simulink model "RobotX_ss_acousticsSingle_Dock_LB_ODOA_T_1024_NewLidarMode"  (R2014a)
settings: Solver=FixedStepDiscrete  StartTime=0.0  StopTime=inf  FixedStep=.25  RelTol=1e-3
undefined symbols (not defined in the file): Com1, Com2, Com3, Com4, DiscIntNeverNeededParam, standard
libraries: xpcseriallib x42, simulink x19, slrtlib x7, dspmtrx3 x2, speedgoatlib x2, speedgoatlib_IO102 x1
(part 4 of 7)

== matlab function RobotX_ss_acousticsSingle_Dock_LB_ODOA_T_1024_NewLidarMode/Main FSM/Start//Speedgate/Aim/LLA to NED ==
  data: LLA input; GoalNED output; NED_origin input
function GoalNED = LLA2NEDfun(LLA,NED_origin)
%Written by Anderson Lebbad on September 20, 2014
%Last edited by:
%
%This function converts a target Latitude, Longitude, Altitude (LLA) point
%into North, East, Down (NED) coordinates

%First convert to earth centered, earth fixed frame
GoalECEF = lla2ecef([LLA*(pi/180), 0]');
%Then convert from ECEF to North East Down
GoalNEDvect = ecef2ned(NED_origin'*(pi/180),GoalECEF);
GoalNED = GoalNEDvect(1:2)';


end

function x_ecef = lla2ecef(x_lla)
% LLE2ECEF: Converts from geodetic latitude, longitude, and altitude to earth-centered earth-fixed Cartesian coordinates
% INPUT: latitude phi (rad), longitude lambda (rad), altitude h (m)
% OUTPUT: [x, y, z]' (m) earth-centered earth-fixed Cartesian coordinates
    a = 6378137; % equatorial radius of ellipsoid (semi-major axis) (m)
    b = 6356752; % polar axis radius of ellipsoid (semi-minor axis) (m)

    phi = x_lla(1);
    lambda = x_lla(2);
    h = x_lla(3);
    
    % auxiliar quantities f, e, and N
    f = (a-b)/a;
    e = f*(2-f);
    N = a/sqrt(1-(e*sin(phi))^2);
    x_ecef = [(N+h)*cos(phi)*cos(lambda); (N+h)*cos(phi)*sin(lambda); (N*(1-e^2)+h)*sin(phi)];
end

function [x_ned] = ecef2ned(ned_lla, x_ecef)
% ECEF2NED Converts from earth-centered, earth-fixed Cartesian coordinates to tangent plane
% INPUT:
% 1) x_ecef=[x,y,z]' (m) earth-centered, earth-fixed Cartesian coordinates
% 2) ned_lla=[phi,lambda]' consiting of latitude phi (rad), longitude lambda (rad) of NED origin
% OUTPUT:
% 1) x_ned=[x,y,z]' (m) in NED coordinate system with the origin [phi,lambda]'

    phi = ned_lla(1);
    lambda = ned_lla(2);

    % transformation  matrix
    T = [-sin(phi)*cos(lambda) -sin(phi)*sin(lambda)  cos(phi)
         -sin(lambda)           cos(lambda)           0
          cos(phi)*cos(lambda)   cos(phi)*sin(lambda)  sin(phi)];

     x_ned = T*(x_ecef-lla2ecef([phi, lambda, 0]')); % convert to NED
     x_ned(3) = -x_ned(3);
end

== matlab function RobotX_ss_acousticsSingle_Dock_LB_ODOA_T_1024_NewLidarMode/Main FSM/Termination/CalcTimes ==
  data: pts input; u input; Data output
function Data = calcTimes(pts, u)
%Written by Anderson Lebbad on August 9, 2014
%Last Edited: Dylan DeGaetano September 1, 2014

%Calculates times for the boat to get to points for a trajectory, and
%formats Data for communication

%Initialize
Data = zeros(24,1);
traj = zeros(8,3);
traj(:,1:2) = pts;



for k = 2:8
    %Calculate distance to travel from last point
    distTravel = sqrt(sum((pts(k-1,:)-pts(k,:)).^2));
    %Assume 1m per second speed
    traj(k,3) = traj(k-1,3) + distTravel;
    %Add time based off initial velocity to get to first point past initial
    if k == 2
        traj(k,3) = traj(k,3) + 2.5*abs(2-u);
    end
end


%Output Data
for i=1:8
    for j = 1:3
        Data(3*(i-1)+j) = traj(i,j);
    end
end

== matlab function RobotX_ss_acousticsSingle_Dock_LB_ODOA_T_1024_NewLidarMode/Main FSM/Termination/LLA to NED ==
  data: Course input; GoalLLA input; GoalNED output; NED_origin input
function GoalNED = LLA2NEDfun(Course,GoalLLA,NED_origin)
%Written by Anderson Lebbad on September 20, 2014
%Last edited by:
%
%This function converts a target Latitude, Longitude, Altitude (LLA) point
%into North, East, Down (NED) coordinates

%First convert to earth centered, earth fixed frame
GoalECEF1 = lla2ecef([GoalLLA(1,:)*(pi/180), 0]');
%Then convert from ECEF to North East Down
GoalNEDvect1 = ecef2ned(NED_origin'*(pi/180),GoalECEF1);
GoalNED1 = GoalNEDvect1(1:2)';

%First convert to earth centered, earth fixed frame
GoalECEF2 = lla2ecef([GoalLLA(2,:)*(pi/180), 0]');
%Then convert from ECEF to North East Down
GoalNEDvect2 = ecef2ned(NED_origin'*(pi/180),GoalECEF2);
GoalNED2 = GoalNEDvect2(1:2)';

GoalNED = (GoalNED1 + GoalNED2) / 2;

if Course == uint8('T')
    GoalNED = GoalLLA(1,:);
end

end

function x_ecef = lla2ecef(x_lla)
% LLE2ECEF: Converts from geodetic latitude, longitude, and altitude to earth-centered earth-fixed Cartesian coordinates
% INPUT: latitude phi (rad), longitude lambda (rad), altitude h (m)
% OUTPUT: [x, y, z]' (m) earth-centered earth-fixed Cartesian coordinates
    a = 6378137; % equatorial radius of ellipsoid (semi-major axis) (m)
    b = 6356752; % polar axis radius of ellipsoid (semi-minor axis) (m)

    phi = x_lla(1);
    lambda = x_lla(2);
    h = x_lla(3);
    
    % auxiliar quantities f, e, and N
    f = (a-b)/a;
    e = f*(2-f);
    N = a/sqrt(1-(e*sin(phi))^2);
    x_ecef = [(N+h)*cos(phi)*cos(lambda); (N+h)*cos(phi)*sin(lambda); (N*(1-e^2)+h)*sin(phi)];
end

function [x_ned] = ecef2ned(ned_lla, x_ecef)
% ECEF2NED Converts from earth-centered, earth-fixed Cartesian coordinates to tangent plane
% INPUT:
% 1) x_ecef=[x,y,z]' (m) earth-centered, earth-fixed Cartesian coordinates
% 2) ned_lla=[phi,lambda]' consiting of latitude phi (rad), longitude lambda (rad) of NED origin
% OUTPUT:
% 1) x_ned=[x,y,z]' (m) in NED coordinate system with the origin [phi,lambda]'

    phi = ned_lla(1);
    lambda = ned_lla(2);

    % transformation  matrix
    T = [-sin(phi)*cos(lambda) -sin(phi)*sin(lambda)  cos(phi)
         -sin(lambda)           cos(lambda)           0
          cos(phi)*cos(lambda)   cos(phi)*sin(lambda)  sin(phi)];

     x_ned = T*(x_ecef-lla2ecef([phi, lambda, 0]')); % convert to NED
     x_ned(3) = -x_ned(3);
end

== system RobotX_ss_acousticsSingle_Dock_LB_ODOA_T_1024_NewLidarMode/Sensors/1020 Comms/ Raspberry Pi LCM (Navigation) ==
  LCM Input : Inport
  ASCII Decode 6 : xpcseriallib/ASCII Decode   format=P1:%f P2:%f P3:%f V1:%f V2:%f V3:%f E1:%f E2:%f E3:%f Lat:%f Long:%f Pt1:%f Pt2:%f St1:%f St2:%f Start:%f Elapsed:%f RC:%d Deploy:%u Elapsed:%f Bearing1:%f Bearing2:%f Range:%f X_Pos:%f Y_Pos:%f \r\n  nvars=25  vartypes={}
  Bus Creator1 : BusCreator  Inputs=3
  Bus Creator2 : BusCreator  Inputs=3
  Bus Creator3 : BusCreator  Inputs=3
  Bus Creator4 : BusCreator  Inputs=9
  Bus Creator5 : BusCreator  Inputs=2
  Bus Creator6 : BusCreator  Inputs=2
  Bus Creator7 : BusCreator  Inputs=2
  Bus Creator8 : BusCreator  Inputs=7
  Data Type Conversion : DataTypeConversion  OutDataTypeStr=double
  FIFO ASCII read 1 : xpcseriallib/FIFO ASCII read   header={'P1:'}  term=[13 10]  hold=Zero output if no new data  enable=off  maxsize=2000  outputtype=8 bit uint null terminated  sampletime=-1
  LCM Output : Outport
  Acou LCM : Outport  Port=2
  wires:
  LCM Input/1 -> FIFO ASCII read 1/1
  FIFO ASCII read 1/1 -> ASCII Decode 6/1
  Bus Creator4/1 -> LCM Output/1  "Navigation Message"
  ASCII Decode 6/1 -> Bus Creator1/1  "X"
  ASCII Decode 6/2 -> Bus Creator1/2  "Y"
  ASCII Decode 6/3 -> Bus Creator1/3  "Psi"
  Bus Creator1/1 -> Bus Creator4/1  "Pose"
  ASCII Decode 6/4 -> Bus Creator2/1  "u"
  ASCII Decode 6/5 -> Bus Creator2/2  "v"
  Bus Creator2/1 -> Bus Creator4/2  "Velocity"
  ASCII Decode 6/7 -> Bus Creator3/1  "Roll"
  ASCII Decode 6/8 -> Bus Creator3/2  "Pitch"
  ASCII Decode 6/9 -> Bus Creator3/3  "Yaw"
  Bus Creator3/1 -> Bus Creator4/3  "Euler"
  Bus Creator5/1 -> Bus Creator4/5  "Port"
  Bus Creator6/1 -> Bus Creator4/6  "Stbd"
  ASCII Decode 6/14 -> Bus Creator6/1  "StThrust"
  ASCII Decode 6/15 -> Bus Creator6/2  "StAzimuth"
  ASCII Decode 6/12 -> Bus Creator5/1  "PtThrust"
  ASCII Decode 6/13 -> Bus Creator5/2  "PtAzimuth"
  ASCII Decode 6/16 -> Bus Creator4/7  "Start"
  ASCII Decode 6/17 -> Bus Creator4/8  "Elapsed"
  ASCII Decode 6/18 -> Data Type Conversion/1  "On/Off/RC/Auto"
  Data Type Conversion/1 -> Bus Creator4/9  "On/Off/RC/Auto"
  ASCII Decode 6/6 -> Bus Creator2/3  "r"
  ASCII Decode 6/10 -> Bus Creator7/1  "Lat"
  ASCII Decode 6/11 -> Bus Creator7/2  "Long"
  Bus Creator7/1 -> Bus Creator4/4  "GPS (LLA)"
  ASCII Decode 6/19 -> Bus Creator8/1  "Deployed"
  ASCII Decode 6/20 -> Bus Creator8/2  "Elapsed Time"
  ASCII Decode 6/21 -> Bus Creator8/3  "Horizontal Bearing"
  ASCII Decode 6/22 -> Bus Creator8/4  "Vertical Bearing"
  ASCII Decode 6/23 -> Bus Creator8/5  "Range"
  ASCII Decode 6/24 -> Bus Creator8/6  "X Pos"
  ASCII Decode 6/25 -> Bus Creator8/7  "Y Pos"
  Bus Creator8/1 -> Acou LCM/1

== system RobotX_ss_acousticsSingle_Dock_LB_ODOA_T_1024_NewLidarMode/Sensors/1020 Comms/Acoustic LCM ==
  LCM Input : Inport
  Bus Creator : BusCreator  Inputs=2
  Bus Creator1 : BusCreator
  Bus Creator2 : BusCreator  Inputs=3
  Bus Selector : BusSelector  OutputSignals=Deployed,Elapsed Time,Horizontal Bearing,Vertical Bearing,Range,X Pos,Y Pos
  LCM Output : Outport
  wires:
  Bus Selector/3 -> Bus Creator/1  "<Horizontal Bearing>"
  Bus Selector/4 -> Bus Creator/2  "<Vertical Bearing>"
  Bus Creator/1 -> Bus Creator1/3  "Bearings"
  Bus Selector/2 -> Bus Creator1/2  "<Elapsed Time>"
  Bus Selector/1 -> Bus Creator1/1  "<Deployed>"
  Bus Creator1/1 -> LCM Output/1  "Acoustic Message"
  LCM Input/1 -> Bus Selector/1
  Bus Selector/5 -> Bus Creator2/1  "<Range>"
  Bus Selector/6 -> Bus Creator2/2  "<X Pos>"
  Bus Selector/7 -> Bus Creator2/3  "<Y Pos>"
  Bus Creator2/1 -> Bus Creator1/4  "Pose Estimate"

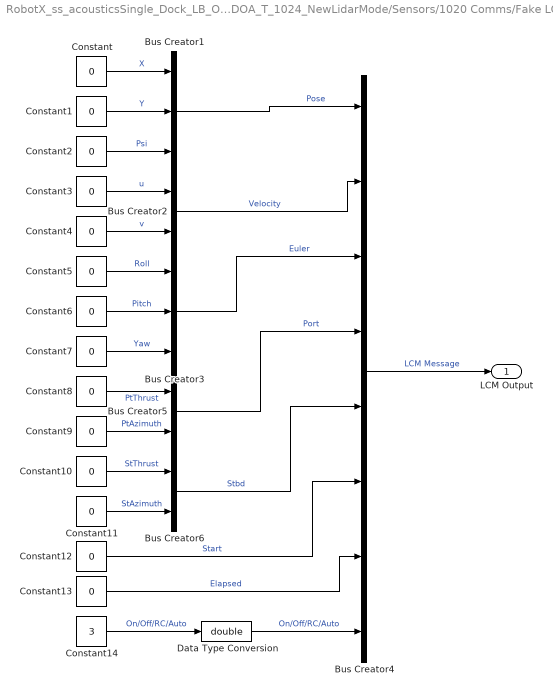
== system RobotX_ss_acousticsSingle_Dock_LB_ODOA_T_1024_NewLidarMode/Sensors/1020 Comms/Fake LCM ==
  Bus Creator1 : BusCreator  Inputs=3
  Bus Creator2 : BusCreator  Inputs=2
  Bus Creator3 : BusCreator  Inputs=3
  Bus Creator4 : BusCreator  Inputs=8
  Bus Creator5 : BusCreator  Inputs=2
  Bus Creator6 : BusCreator  Inputs=2
  Constant{,1..13} (14 alike) : Constant  Value=0
  Constant14 : Constant  Value=3
  Data Type Conversion : DataTypeConversion  OutDataTypeStr=double
  LCM Output : Outport
  wires:
  Bus Creator4/1 -> LCM Output/1  "LCM Message"
  Constant/1 -> Bus Creator1/1  "X"
  Constant1/1 -> Bus Creator1/2  "Y"
  Constant2/1 -> Bus Creator1/3  "Psi"
  Bus Creator1/1 -> Bus Creator4/1  "Pose"
  Constant3/1 -> Bus Creator2/1  "u"
  Constant4/1 -> Bus Creator2/2  "v"
  Bus Creator2/1 -> Bus Creator4/2  "Velocity"
  Constant5/1 -> Bus Creator3/1  "Roll"
  Constant6/1 -> Bus Creator3/2  "Pitch"
  Constant7/1 -> Bus Creator3/3  "Yaw"
  Bus Creator3/1 -> Bus Creator4/3  "Euler"
  Bus Creator5/1 -> Bus Creator4/4  "Port"
  Bus Creator6/1 -> Bus Creator4/5  "Stbd"
  Constant10/1 -> Bus Creator6/1  "StThrust"
  Constant11/1 -> Bus Creator6/2  "StAzimuth"
  Constant8/1 -> Bus Creator5/1  "PtThrust"
  Constant9/1 -> Bus Creator5/2  "PtAzimuth"
  Constant12/1 -> Bus Creator4/6  "Start"
  Constant13/1 -> Bus Creator4/7  "Elapsed"
  Constant14/1 -> Data Type Conversion/1  "On/Off/RC/Auto"
  Data Type Conversion/1 -> Bus Creator4/8  "On/Off/RC/Auto"

== system RobotX_ss_acousticsSingle_Dock_LB_ODOA_T_1024_NewLidarMode/Sensors/1020 Comms/LIDAR Panda ==
  LIDAR Panda In : Inport
  ASCII Decode 2 : xpcseriallib/ASCII Decode   format=A:%d B:%d C:%d E:%d F:%d G:%d H:%d I:%d J:%d K:%d L:%d M:%d N:%d O:%d P:%d Q:%d R:%d S:%d T:%d U:%d V:%d W:%d X:%d C1:%d C2:%d C3:%d C4:%d P1:%f P2:%f P3:%f P4:%f I1:%d I2:%d I3:%d I4:%d \r\n  nvars=36  vartypes={}
  Bus Creator1 : BusCreator  Inputs=2
  Bus Creator2 : BusCreator  Inputs=3
  Bus Creator3 : BusCreator  Inputs=2
  Data Type Conversion{,1..3} (4 alike) : DataTypeConversion  OutDataTypeStr=double
  "FIFO ASCII read " : xpcseriallib/FIFO ASCII read   header={'A:'}  term=[13 10]  hold=Zero output if no new data  enable=off  maxsize=1024  outputtype=8 bit uint null terminated  sampletime=-1
  Mux : Mux  Inputs=12
  Mux1 : Mux
  Mux2 : Mux  Inputs=12
  Mux3 : Mux
  Mux4 : Mux
  LIDAR Panda Out : Outport
  wires:
  LIDAR Panda In/1 -> "FIFO ASCII read "/1
  "FIFO ASCII read "/1 -> ASCII Decode 2/1
  ASCII Decode 2/3 -> Mux/3  "Distance"
  ASCII Decode 2/2 -> Mux/2  "Color ID"
  ASCII Decode 2/4 -> Mux/4  "Angle"
  ASCII Decode 2/1 -> Mux/1  "Probability"
  ASCII Decode 2/7 -> Mux/7
  ASCII Decode 2/10 -> Mux/10
  ASCII Decode 2/11 -> Mux/11
  ASCII Decode 2/6 -> Mux/6
  ASCII Decode 2/8 -> Mux/8
  ASCII Decode 2/9 -> Mux/9
  ASCII Decode 2/12 -> Mux/12
  ASCII Decode 2/5 -> Mux/5
  ASCII Decode 2/13 -> Mux2/1
  ASCII Decode 2/15 -> Mux2/3
  ASCII Decode 2/22 -> Mux2/10
  ASCII Decode 2/23 -> Mux2/11
  ASCII Decode 2/17 -> Mux2/5
  ASCII Decode 2/18 -> Mux2/6
  ASCII Decode 2/14 -> Mux2/2
  ASCII Decode 2/24 -> Mux2/12
  ASCII Decode 2/20 -> Mux2/8
  ASCII Decode 2/19 -> Mux2/7
  ASCII Decode 2/21 -> Mux2/9
  ASCII Decode 2/16 -> Mux2/4
  ASCII Decode 2/25 -> Mux1/1
  ASCII Decode 2/28 -> Mux1/4
  ASCII Decode 2/26 -> Mux1/2
  ASCII Decode 2/27 -> Mux1/3
  ASCII Decode 2/30 -> Mux3/2
  ASCII Decode 2/31 -> Mux3/3
  ASCII Decode 2/32 -> Mux3/4
  ASCII Decode 2/29 -> Mux3/1
  ASCII Decode 2/36 -> Mux4/4
  ASCII Decode 2/34 -> Mux4/2
  ASCII Decode 2/35 -> Mux4/3
  ASCII Decode 2/33 -> Mux4/1
  Mux/1 -> Data Type Conversion/1  "Distances"
  Mux2/1 -> Data Type Conversion1/1  "Angles"
  Mux1/1 -> Data Type Conversion2/1  "Color"
  Mux3/1 -> Bus Creator2/2  "Probability"
  Mux4/1 -> Data Type Conversion3/1  "idx"
  Bus Creator1/1 -> Bus Creator3/1  "Landmarks"
  Bus Creator2/1 -> Bus Creator3/2  "Color data"
  Bus Creator3/1 -> LIDAR Panda Out/1
  Data Type Conversion/1 -> Bus Creator1/1  "Distances"
  Data Type Conversion1/1 -> Bus Creator1/2  "Angles"
  Data Type Conversion2/1 -> Bus Creator2/1  "Color"
  Data Type Conversion3/1 -> Bus Creator2/3  "Color"

== system RobotX_ss_acousticsSingle_Dock_LB_ODOA_T_1024_NewLidarMode/Sensors/1020 Comms/Subsystem ==
  Bus Creator : BusCreator  Inputs=3
  Bus Creator1 : BusCreator  Inputs=2
  Bus Creator2 : BusCreator  Inputs=2
  Constant : Constant  Value=zeros(12,1)
  Constant1 : Constant  Value=zeros(12,1)
  Constant2 : Constant  Value=zeros(4,1)
  Constant3 : Constant  Value=zeros(4,1)
  Constant4 : Constant  Value=zeros(4,1)
  Fake Panda : Outport
  wires:
  Constant/1 -> Bus Creator1/1  "Distances"
  Constant1/1 -> Bus Creator1/2  "Angles"
  Constant2/1 -> Bus Creator/1  "Color"
  Constant3/1 -> Bus Creator/2  "Probability"
  Constant4/1 -> Bus Creator/3  "idx"
  Bus Creator1/1 -> Bus Creator2/1  "Landmarks"
  Bus Creator/1 -> Bus Creator2/2  "Color data"
  Bus Creator2/1 -> Fake Panda/1  "Lidar Data Input"

== system RobotX_ss_acousticsSingle_Dock_LB_ODOA_T_1024_NewLidarMode/Sensors/1020 Comms/data log ==
  Sensors signal : Inport
  Bus Selector3 : BusSelector  OutputSignals=Navigation Message,Lidar Data Input,Acoustic Message
  Bus to Vector : BusToVector
  Bus to Vector1 : BusToVector
  Bus to Vector2 : BusToVector
  Read : DataStoreRead  DataStoreName=PingPose
  Scope 1 : slrtlib/Displays and Logging/Scope   scopeno=3  scopetype=File  autostart=on  viewmode=Graphical redraw  formatstr='%15.6f'  grid=on  ylimits=[0,0]  nosamples=28800  noprepostsamples=0  interleave=1  triggermode=FreeRun  triggersignal=1  trigsignalfromport=off  triggerlevel=0.0  triggerslope=Either  triggerscope=1  triggersample=0  filename=LM1_<%%%>.dat  mode=Lazy  writesize=5120  autorestart=on  dynamicfilemode=on  maxwritefilesize=512*1024^2
  Scope 2 : slrtlib/Displays and Logging/Scope   scopeno=1  scopetype=File  autostart=on  viewmode=Graphical redraw  formatstr='%15.6f'  grid=on  ylimits=[0,0]  nosamples=28800  noprepostsamples=0  interleave=1  triggermode=FreeRun  triggersignal=1  trigsignalfromport=off  triggerlevel=0.0  triggerslope=Either  triggerscope=1  triggersample=0  filename=NAV1_<%%%>.dat  mode=Lazy  writesize=5120  autorestart=on  dynamicfilemode=on  maxwritefilesize=512*1024^2
  Scope 3 : slrtlib/Displays and Logging/Scope   scopeno=2  scopetype=File  autostart=on  viewmode=Graphical redraw  formatstr='%15.6f'  grid=on  ylimits=[0,0]  nosamples=28800  noprepostsamples=0  interleave=1  triggermode=FreeRun  triggersignal=1  trigsignalfromport=off  triggerlevel=0.0  triggerslope=Either  triggerscope=1  triggersample=0  filename=ACO1_<%%%>.dat  mode=Lazy  writesize=5120  autorestart=on  dynamicfilemode=on  maxwritefilesize=512*1024^2
  Scope 4 : slrtlib/Displays and Logging/Scope   scopeno=4  scopetype=File  autostart=on  viewmode=Graphical redraw  formatstr='%15.6f'  grid=on  ylimits=[0,0]  nosamples=28800  noprepostsamples=0  interleave=1  triggermode=FreeRun  triggersignal=1  trigsignalfromport=off  triggerlevel=0.0  triggerslope=Either  triggerscope=1  triggersample=0  filename=pPos_<%%%>.dat  mode=Lazy  writesize=5120  autorestart=on  dynamicfilemode=on  maxwritefilesize=512*1024^2
  wires:
  Sensors signal/1 -> Bus Selector3/1
  Bus to Vector/1 -> Scope 2/1
  Bus Selector3/1 -> Bus to Vector/1  "<Navigation Message>"
  Bus to Vector1/1 -> Scope 1/1
  Bus to Vector2/1 -> Scope 3/1
  Bus Selector3/3 -> Bus to Vector2/1  "<Acoustic Message>"
  Bus Selector3/2 -> Bus to Vector1/1  "<Lidar Data Input>"
  Read/1 -> Scope 4/1

== system RobotX_ss_acousticsSingle_Dock_LB_ODOA_T_1024_NewLidarMode/Sensors/1024 Comms New LIDAR Mode/ Raspberry Pi LCM (Acoustic) ==
  LCM Input : Inport
  ASCII Decode 6 : xpcseriallib/ASCII Decode   format=Deploy:%1u, Elapsed:%g, Bearing1:%g Bearing2:%g \r\n  nvars=4  vartypes={}
  Bus Creator : BusCreator  Inputs=2
  Bus Creator1 : BusCreator  Inputs=3
  FIFO ASCII read 1 : xpcseriallib/FIFO ASCII read   header={'Deploy:'}  term=[13 10]  hold=Zero output if no new data  enable=off  maxsize=1024  outputtype=8 bit uint null terminated  sampletime=-1
  LCM Output : Outport
  wires:
  LCM Input/1 -> FIFO ASCII read 1/1
  FIFO ASCII read 1/1 -> ASCII Decode 6/1
  ASCII Decode 6/3 -> Bus Creator/1  "Horizontal Bearing"
  ASCII Decode 6/4 -> Bus Creator/2  "Vertical Bearing"
  Bus Creator/1 -> Bus Creator1/3  "Bearings"
  ASCII Decode 6/2 -> Bus Creator1/2  "Elapsed Time"
  ASCII Decode 6/1 -> Bus Creator1/1  "Deployed"
  Bus Creator1/1 -> LCM Output/1  "Acoustic Message"

== system RobotX_ss_acousticsSingle_Dock_LB_ODOA_T_1024_NewLidarMode/Sensors/1024 Comms New LIDAR Mode/ Raspberry Pi LCM (Navigation and Acoustics) ==
  LCM Input : Inport
  ASCII Decode 6 : xpcseriallib/ASCII Decode   format=P1:%f P2:%f P3:%f V1:%f V2:%f V3:%f E1:%f E2:%f E3:%f Pt1:%f Pt2:%f St1:%f St2:%f Start:%f Elapsed:%f RC:%d Deploy:%u, Elapsed:%g, Bearing1:%g Bearing2:%g \r\n  nvars=22  vartypes={}
  Bus Creator{,5..7} (4 alike) : BusCreator  Inputs=2
  Bus Creator{1..3,8} (4 alike) : BusCreator  Inputs=3
  Bus Creator4 : BusCreator  Inputs=9
  Data Type Conversion : DataTypeConversion  OutDataTypeStr=double
  FIFO ASCII read 1 : xpcseriallib/FIFO ASCII read   header={'P1:'}  term=[13 10]  hold=Zero output if no new data  enable=off  maxsize=2048  outputtype=8 bit uint null terminated  sampletime=-1
  Navigation LCM : Outport
  Acoustic LCM : Outport  Port=2
  wires:
  LCM Input/1 -> FIFO ASCII read 1/1
  FIFO ASCII read 1/1 -> ASCII Decode 6/1
  Bus Creator4/1 -> Navigation LCM/1  "Navigation Message"
  ASCII Decode 6/1 -> Bus Creator1/1  "X"
  ASCII Decode 6/2 -> Bus Creator1/2  "Y"
  ASCII Decode 6/3 -> Bus Creator1/3  "Psi"
  Bus Creator1/1 -> Bus Creator4/1  "Pose"
  ASCII Decode 6/4 -> Bus Creator2/1  "u"
  ASCII Decode 6/5 -> Bus Creator2/2  "v"
  Bus Creator2/1 -> Bus Creator4/2  "Velocity"
  ASCII Decode 6/7 -> Bus Creator3/1  "Roll"
  ASCII Decode 6/8 -> Bus Creator3/2  "Pitch"
  ASCII Decode 6/9 -> Bus Creator3/3  "Yaw"
  Bus Creator3/1 -> Bus Creator4/3  "Euler"
  Bus Creator5/1 -> Bus Creator4/5  "Port"
  Bus Creator6/1 -> Bus Creator4/6  "Stbd"
  ASCII Decode 6/14 -> Bus Creator6/1  "StThrust"
  ASCII Decode 6/15 -> Bus Creator6/2  "StAzimuth"
  ASCII Decode 6/12 -> Bus Creator5/1  "PtThrust"
  ASCII Decode 6/13 -> Bus Creator5/2  "PtAzimuth"
  ASCII Decode 6/16 -> Bus Creator4/7  "Start"
  ASCII Decode 6/17 -> Bus Creator4/8  "Elapsed"
  ASCII Decode 6/18 -> Data Type Conversion/1  "On/Off/RC/Auto"
  Data Type Conversion/1 -> Bus Creator4/9  "On/Off/RC/Auto"
  ASCII Decode 6/6 -> Bus Creator2/3  "r"
  ASCII Decode 6/10 -> Bus Creator7/1  "Lat"
  ASCII Decode 6/11 -> Bus Creator7/2  "Long"
  Bus Creator7/1 -> Bus Creator4/4  "GPS (LLA)"
  ASCII Decode 6/21 -> Bus Creator/1  "Horizontal Bearing"
  ASCII Decode 6/22 -> Bus Creator/2  "Vertical Bearing"
  Bus Creator/1 -> Bus Creator8/3  "Bearings"
  ASCII Decode 6/20 -> Bus Creator8/2  "Elapsed Time"
  ASCII Decode 6/19 -> Bus Creator8/1  "Deployed"
  Bus Creator8/1 -> Acoustic LCM/1  "Acoustic Message"

== system RobotX_ss_acousticsSingle_Dock_LB_ODOA_T_1024_NewLidarMode/Sensors/1024 Comms New LIDAR Mode/ Raspberry Pi LCM (Navigation) ==
  LCM Input : Inport
  ASCII Decode 6 : xpcseriallib/ASCII Decode   format=P1:%f P2:%f P3:%f V1:%f V2:%f V3:%f E1:%f E2:%f E3:%f Lat:%f Long:%f Pt1:%f Pt2:%f St1:%f St2:%f Start:%f Elapsed:%f RC:%d Deploy:%u Elapsed:%f Bearing1:%f Bearing2:%f Range:%f X_Pos:%f Y_Pos:%f Depth:%f \r\n  nvars=26  vartypes={}
  Bus Creator1 : BusCreator  Inputs=3
  Bus Creator2 : BusCreator  Inputs=3
  Bus Creator3 : BusCreator  Inputs=3
  Bus Creator4 : BusCreator  Inputs=9
  Bus Creator5 : BusCreator  Inputs=2
  Bus Creator6 : BusCreator  Inputs=2
  Bus Creator7 : BusCreator  Inputs=2
  Bus Creator8 : BusCreator  Inputs=8
  Data Type Conversion : DataTypeConversion  OutDataTypeStr=double
  FIFO ASCII read 1 : xpcseriallib/FIFO ASCII read   header={'P1:'}  term=[13 10]  hold=Zero output if no new data  enable=off  maxsize=2000  outputtype=8 bit uint null terminated  sampletime=-1
  LCM Output : Outport
  Acou LCM : Outport  Port=2
  wires:
  LCM Input/1 -> FIFO ASCII read 1/1
  FIFO ASCII read 1/1 -> ASCII Decode 6/1
  Bus Creator4/1 -> LCM Output/1  "Navigation Message"
  ASCII Decode 6/1 -> Bus Creator1/1  "X"
  ASCII Decode 6/2 -> Bus Creator1/2  "Y"
  ASCII Decode 6/3 -> Bus Creator1/3  "Psi"
  Bus Creator1/1 -> Bus Creator4/1  "Pose"
  ASCII Decode 6/4 -> Bus Creator2/1  "u"
  ASCII Decode 6/5 -> Bus Creator2/2  "v"
  Bus Creator2/1 -> Bus Creator4/2  "Velocity"
  ASCII Decode 6/7 -> Bus Creator3/1  "Roll"
  ASCII Decode 6/8 -> Bus Creator3/2  "Pitch"
  ASCII Decode 6/9 -> Bus Creator3/3  "Yaw"
  Bus Creator3/1 -> Bus Creator4/3  "Euler"
  Bus Creator5/1 -> Bus Creator4/5  "Port"
  Bus Creator6/1 -> Bus Creator4/6  "Stbd"
  ASCII Decode 6/14 -> Bus Creator6/1  "StThrust"
  ASCII Decode 6/15 -> Bus Creator6/2  "StAzimuth"
  ASCII Decode 6/12 -> Bus Creator5/1  "PtThrust"
  ASCII Decode 6/13 -> Bus Creator5/2  "PtAzimuth"
  ASCII Decode 6/16 -> Bus Creator4/7  "Start"
  ASCII Decode 6/17 -> Bus Creator4/8  "Elapsed"
  ASCII Decode 6/18 -> Data Type Conversion/1  "On/Off/RC/Auto"
  Data Type Conversion/1 -> Bus Creator4/9  "On/Off/RC/Auto"
  ASCII Decode 6/6 -> Bus Creator2/3  "r"
  ASCII Decode 6/10 -> Bus Creator7/1  "Lat"
  ASCII Decode 6/11 -> Bus Creator7/2  "Long"
  Bus Creator7/1 -> Bus Creator4/4  "GPS (LLA)"
  ASCII Decode 6/19 -> Bus Creator8/1  "Deployed"
  ASCII Decode 6/20 -> Bus Creator8/2  "Elapsed Time"
  ASCII Decode 6/21 -> Bus Creator8/3  "Horizontal Bearing"
  ASCII Decode 6/22 -> Bus Creator8/4  "Vertical Bearing"
  ASCII Decode 6/23 -> Bus Creator8/5  "Range"
  ASCII Decode 6/24 -> Bus Creator8/6  "X Pos"
  ASCII Decode 6/25 -> Bus Creator8/7  "Y Pos"
  Bus Creator8/1 -> Acou LCM/1
  ASCII Decode 6/26 -> Bus Creator8/8  "Depth"

== system RobotX_ss_acousticsSingle_Dock_LB_ODOA_T_1024_NewLidarMode/Sensors/1024 Comms New LIDAR Mode/Acoustic LCM ==
  LCM Input : Inport
  Bus Creator : BusCreator  Inputs=2
  Bus Creator1 : BusCreator
  Bus Creator2 : BusCreator
  Bus Selector : BusSelector  OutputSignals=Deployed,Elapsed Time,Horizontal Bearing,Vertical Bearing,Range,X Pos,Y Pos,Depth
  LCM Output : Outport
  wires:
  Bus Selector/3 -> Bus Creator/1  "<Horizontal Bearing>"
  Bus Selector/4 -> Bus Creator/2  "<Vertical Bearing>"
  Bus Creator/1 -> Bus Creator1/3  "Bearings"
  Bus Selector/2 -> Bus Creator1/2  "<Elapsed Time>"
  Bus Selector/1 -> Bus Creator1/1  "<Deployed>"
  Bus Creator1/1 -> LCM Output/1  "Acoustic Message"
  LCM Input/1 -> Bus Selector/1
  Bus Selector/5 -> Bus Creator2/1  "<Range>"
  Bus Selector/6 -> Bus Creator2/2  "<X Pos>"
  Bus Selector/7 -> Bus Creator2/3  "<Y Pos>"
  Bus Creator2/1 -> Bus Creator1/4  "Pose Estimate"
  Bus Selector/8 -> Bus Creator2/4  "<Depth>"

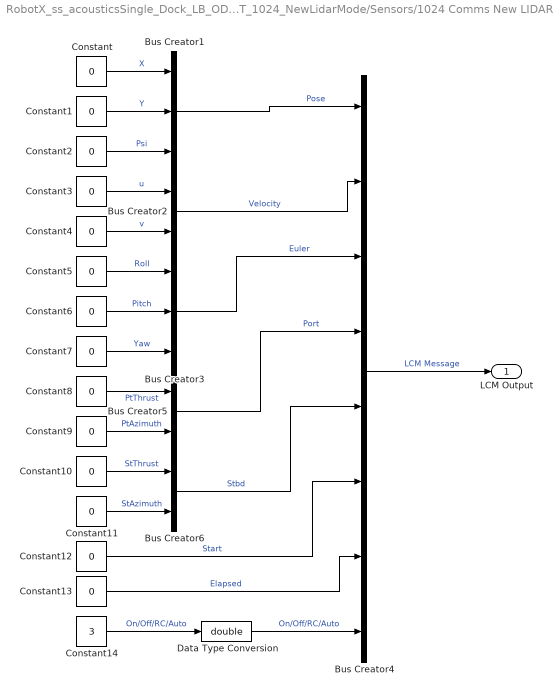
== system RobotX_ss_acousticsSingle_Dock_LB_ODOA_T_1024_NewLidarMode/Sensors/1024 Comms New LIDAR Mode/Fake LCM ==
  Bus Creator1 : BusCreator  Inputs=3
  Bus Creator2 : BusCreator  Inputs=2
  Bus Creator3 : BusCreator  Inputs=3
  Bus Creator4 : BusCreator  Inputs=8
  Bus Creator5 : BusCreator  Inputs=2
  Bus Creator6 : BusCreator  Inputs=2
  Constant{,1..13} (14 alike) : Constant  Value=0
  Constant14 : Constant  Value=3
  Data Type Conversion : DataTypeConversion  OutDataTypeStr=double
  LCM Output : Outport
  wires:
  Bus Creator4/1 -> LCM Output/1  "LCM Message"
  Constant/1 -> Bus Creator1/1  "X"
  Constant1/1 -> Bus Creator1/2  "Y"
  Constant2/1 -> Bus Creator1/3  "Psi"
  Bus Creator1/1 -> Bus Creator4/1  "Pose"
  Constant3/1 -> Bus Creator2/1  "u"
  Constant4/1 -> Bus Creator2/2  "v"
  Bus Creator2/1 -> Bus Creator4/2  "Velocity"
  Constant5/1 -> Bus Creator3/1  "Roll"
  Constant6/1 -> Bus Creator3/2  "Pitch"
  Constant7/1 -> Bus Creator3/3  "Yaw"
  Bus Creator3/1 -> Bus Creator4/3  "Euler"
  Bus Creator5/1 -> Bus Creator4/4  "Port"
  Bus Creator6/1 -> Bus Creator4/5  "Stbd"
  Constant10/1 -> Bus Creator6/1  "StThrust"
  Constant11/1 -> Bus Creator6/2  "StAzimuth"
  Constant8/1 -> Bus Creator5/1  "PtThrust"
  Constant9/1 -> Bus Creator5/2  "PtAzimuth"
  Constant12/1 -> Bus Creator4/6  "Start"
  Constant13/1 -> Bus Creator4/7  "Elapsed"
  Constant14/1 -> Data Type Conversion/1  "On/Off/RC/Auto"
  Data Type Conversion/1 -> Bus Creator4/8  "On/Off/RC/Auto"

== system RobotX_ss_acousticsSingle_Dock_LB_ODOA_T_1024_NewLidarMode/Sensors/1024 Comms New LIDAR Mode/LIDAR Panda ==
  LIDAR Panda In : Inport
  ASCII Decode 2 : xpcseriallib/ASCII Decode   format=A:%d B:%d C:%d E:%d F:%d G:%d H:%d I:%d J:%d K:%d L:%d M:%d N:%d O:%d P:%d Q:%d R:%d S:%d T:%d U:%d V:%d W:%d X:%d C1:%d C2:%d C3:%d C4:%d P1:%f P2:%f P3:%f P4:%f I1:%d I2:%d I3:%d I4:%d \r\n  nvars=36  vartypes={}
  Bus Creator1 : BusCreator  Inputs=2
  Bus Creator2 : BusCreator  Inputs=3
  Bus Creator3 : BusCreator  Inputs=2
  Data Type Conversion{,1..3} (4 alike) : DataTypeConversion  OutDataTypeStr=double
  "FIFO ASCII read " : xpcseriallib/FIFO ASCII read   header={'A:'}  term=[13 10]  hold=Zero output if no new data  enable=off  maxsize=1024  outputtype=8 bit uint null terminated  sampletime=-1
  Mux : Mux  Inputs=12
  Mux1 : Mux
  Mux2 : Mux  Inputs=12
  Mux3 : Mux
  Mux4 : Mux
  LIDAR Panda Out : Outport
  wires:
  LIDAR Panda In/1 -> "FIFO ASCII read "/1
  "FIFO ASCII read "/1 -> ASCII Decode 2/1
  ASCII Decode 2/3 -> Mux/3  "Distance"
  ASCII Decode 2/2 -> Mux/2  "Color ID"
  ASCII Decode 2/4 -> Mux/4  "Angle"
  ASCII Decode 2/1 -> Mux/1  "Probability"
  ASCII Decode 2/7 -> Mux/7
  ASCII Decode 2/10 -> Mux/10
  ASCII Decode 2/11 -> Mux/11
  ASCII Decode 2/6 -> Mux/6
  ASCII Decode 2/8 -> Mux/8
  ASCII Decode 2/9 -> Mux/9
  ASCII Decode 2/12 -> Mux/12
  ASCII Decode 2/5 -> Mux/5
  ASCII Decode 2/13 -> Mux2/1
  ASCII Decode 2/15 -> Mux2/3
  ASCII Decode 2/22 -> Mux2/10
  ASCII Decode 2/23 -> Mux2/11
  ASCII Decode 2/17 -> Mux2/5
  ASCII Decode 2/18 -> Mux2/6
  ASCII Decode 2/14 -> Mux2/2
  ASCII Decode 2/24 -> Mux2/12
  ASCII Decode 2/20 -> Mux2/8
  ASCII Decode 2/19 -> Mux2/7
  ASCII Decode 2/21 -> Mux2/9
  ASCII Decode 2/16 -> Mux2/4
  ASCII Decode 2/25 -> Mux1/1
  ASCII Decode 2/28 -> Mux1/4
  ASCII Decode 2/26 -> Mux1/2
  ASCII Decode 2/27 -> Mux1/3
  ASCII Decode 2/30 -> Mux3/2
  ASCII Decode 2/31 -> Mux3/3
  ASCII Decode 2/32 -> Mux3/4
  ASCII Decode 2/29 -> Mux3/1
  ASCII Decode 2/36 -> Mux4/4
  ASCII Decode 2/34 -> Mux4/2
  ASCII Decode 2/35 -> Mux4/3
  ASCII Decode 2/33 -> Mux4/1
  Mux/1 -> Data Type Conversion/1  "Distances"
  Mux2/1 -> Data Type Conversion1/1  "Angles"
  Mux1/1 -> Data Type Conversion2/1  "Color"
  Mux3/1 -> Bus Creator2/2  "Probability"
  Mux4/1 -> Data Type Conversion3/1  "idx"
  Bus Creator1/1 -> Bus Creator3/1  "Landmarks"
  Bus Creator2/1 -> Bus Creator3/2  "Color data"
  Bus Creator3/1 -> LIDAR Panda Out/1
  Data Type Conversion/1 -> Bus Creator1/1  "Distances"
  Data Type Conversion1/1 -> Bus Creator1/2  "Angles"
  Data Type Conversion2/1 -> Bus Creator2/1  "Color"
  Data Type Conversion3/1 -> Bus Creator2/3  "idx"

== system RobotX_ss_acousticsSingle_Dock_LB_ODOA_T_1024_NewLidarMode/Sensors/1024 Comms New LIDAR Mode/Lidar Send ==
  Parameters : Inport
  ASCII Encode 2 : xpcseriallib/ASCII Encode   format=SGTask:%d \r\n  nvars=1  maxlength=128  vartypes={ 'double' }
  Bus Selector1 : BusSelector  OutputSignals=Main Task
  Data Store Read : DataStoreRead  DataStoreName=cameraOnly
  MATLAB Function : MATLAB Function  TreatAsAtomicUnit=on
  Read : DataStoreRead  DataStoreName=symbol
  Serial Send : Outport
  wires:
  Parameters/1 -> Bus Selector1/1
  Bus Selector1/1 -> MATLAB Function/2(MainMode)  "<Main Task>"
  Read/1 -> MATLAB Function/1(symbol)
  MATLAB Function/1(LidarMode) -> ASCII Encode 2/1
  ASCII Encode 2/1 -> Serial Send/1
  Data Store Read/1 -> MATLAB Function/3(cameraOnly)

== system RobotX_ss_acousticsSingle_Dock_LB_ODOA_T_1024_NewLidarMode/Sensors/1024 Comms New LIDAR Mode/Message Selector ==
  Parameters : Inport
  Real Time : Inport  Port=2
  Bus Selector : BusSelector  OutputSignals=Main Task
  HRT Message : Subsystem
  HRTLIT Message : Subsystem
  HRTSEA Message : Subsystem
  MATLAB Function : MATLAB Function  TreatAsAtomicUnit=on
  Multiport Switch : MultiPortSwitch
  Message : Outport
  wires:
  MATLAB Function/1(messageNumber) -> Multiport Switch/1
  HRT Message/1(HRT Message) -> Multiport Switch/2
  HRTSEA Message/1(HRTSEA Message) -> Multiport Switch/3
  HRTLIT Message/1(HRTLIT Message) -> Multiport Switch/4
  Multiport Switch/1 -> Message/1
  Parameters/1 -> HRTLIT Message/1(Parameters), HRTSEA Message/1(Parameters), HRT Message/1(Parameters), Bus Selector/1
  Bus Selector/1 -> MATLAB Function/1(taskNumber)  "<Main Task>"
  Real Time/1 -> HRTSEA Message/2(Time), HRT Message/2(Time), HRTLIT Message/2(Time)

== system RobotX_ss_acousticsSingle_Dock_LB_ODOA_T_1024_NewLidarMode/Sensors/1024 Comms New LIDAR Mode/Pi Nav Send ==
  Parameters : Inport
  ASCII Encode 3 : xpcseriallib/ASCII Encode   format="{\"Valid\":%d, \"Mode\":%d, \"Length\":%d, \"Activate\":%d, \"Waypoints\":[%f, %f, %f, %f, %f, %f, %f, %f, %f, %f, %f, %f, %f, %f, %f, %f, %f, %f, %f, %f, %f, %f, %f, %f]} \\r\\n"  nvars=28  maxlength=1000  vartypes={ 'double' }
  Bus Selector : BusSelector  OutputSignals=Outputs.Navigation Outputs.Valid,Outputs.Navigation Outputs.Control Mode,Outputs.Navigation Outputs.Data,Outputs.Acoustic Active
  Data Update1 : MATLAB Function  Commented=on  TreatAsAtomicUnit=on
  Data Update2 : MATLAB Function  TreatAsAtomicUnit=on
  LCM Complete Encode : xpcseriallib/ASCII Encode   Commented=on  format="{\"Valid\":%d, \"Mode\":%d, \"Length\":%d, \"Activate\":%d, \"Waypoints\":[%f, %f, %f, %f, %f, %f, %f, %f, %f, %f, %f, %f, %f, %f, %f, %f, %f, %f, %f, %f, %f, %f, %f, %f]} \\r\\n"  nvars=28  maxlength=1000  vartypes={ 'double' }
  Serial Send : Outport
  wires:
  Parameters/1 -> Bus Selector/1
  ASCII Encode 3/1 -> Serial Send/1
  Bus Selector/1 -> Data Update2/1(Valid)  "<Valid>"
  Bus Selector/2 -> Data Update2/2(ControlMode)  "<Control Mode>"
  Bus Selector/3 -> Data Update2/3(Data)  "<Data>"
  Data Update2/21(D17) -> ASCII Encode 3/21
  Data Update2/20(D16) -> ASCII Encode 3/20
  Data Update2/19(D15) -> ASCII Encode 3/19
  Data Update2/4(A) -> ASCII Encode 3/4
  Data Update2/2(C) -> ASCII Encode 3/2
  Data Update2/18(D14) -> ASCII Encode 3/18
  Data Update2/16(D12) -> ASCII Encode 3/16
  Data Update2/7(D3) -> ASCII Encode 3/7
  Data Update2/6(D2) -> ASCII Encode 3/6
  Data Update2/5(D1) -> ASCII Encode 3/5
  Data Update2/17(D13) -> ASCII Encode 3/17
  Data Update2/9(D5) -> ASCII Encode 3/9
  Data Update2/10(D6) -> ASCII Encode 3/10
  Data Update2/24(D20) -> ASCII Encode 3/24
  Data Update2/23(D19) -> ASCII Encode 3/23
  Data Update2/28(D24) -> ASCII Encode 3/28
  Data Update2/26(D22) -> ASCII Encode 3/26
  Data Update2/25(D21) -> ASCII Encode 3/25
  Data Update2/3(L) -> ASCII Encode 3/3
  Data Update2/27(D23) -> ASCII Encode 3/27
  Data Update2/8(D4) -> ASCII Encode 3/8
  Data Update2/11(D7) -> ASCII Encode 3/11
  Data Update2/13(D9) -> ASCII Encode 3/13
  Data Update2/12(D8) -> ASCII Encode 3/12
  Data Update2/14(D10) -> ASCII Encode 3/14
  Data Update2/22(D18) -> ASCII Encode 3/22
  Data Update2/15(D11) -> ASCII Encode 3/15
  Bus Selector/4 -> Data Update2/4(Activate)  "<Acoustic Active>"
  Data Update2/1(V) -> ASCII Encode 3/1
  Data Update1/1(V) -> LCM Complete Encode/1
  Data Update1/2(C) -> LCM Complete Encode/2
  Data Update1/6(D2) -> LCM Complete Encode/6
  Data Update1/7(D3) -> LCM Complete Encode/7
  Data Update1/8(D4) -> LCM Complete Encode/8
  Data Update1/5(D1) -> LCM Complete Encode/5
  Data Update1/9(D5) -> LCM Complete Encode/9
  Data Update1/10(D6) -> LCM Complete Encode/10
  Data Update1/11(D7) -> LCM Complete Encode/11
  Data Update1/12(D8) -> LCM Complete Encode/12
  Data Update1/13(D9) -> LCM Complete Encode/13
  Data Update1/18(D14) -> LCM Complete Encode/18
  Data Update1/15(D11) -> LCM Complete Encode/15
  Data Update1/20(D16) -> LCM Complete Encode/20
  Data Update1/21(D17) -> LCM Complete Encode/21
  Data Update1/19(D15) -> LCM Complete Encode/19
  Data Update1/14(D10) -> LCM Complete Encode/14
  Data Update1/16(D12) -> LCM Complete Encode/16
  Data Update1/22(D18) -> LCM Complete Encode/22
  Data Update1/23(D19) -> LCM Complete Encode/23
  Data Update1/24(D20) -> LCM Complete Encode/24
  Data Update1/25(D21) -> LCM Complete Encode/25
  Data Update1/27(D23) -> LCM Complete Encode/27
  Data Update1/26(D22) -> LCM Complete Encode/26
  Data Update1/28(D24) -> LCM Complete Encode/28
  Data Update1/3(L) -> LCM Complete Encode/3
  Data Update1/4(A) -> LCM Complete Encode/4
  Data Update1/17(D13) -> LCM Complete Encode/17

== system RobotX_ss_acousticsSingle_Dock_LB_ODOA_T_1024_NewLidarMode/Sensors/1024 Comms New LIDAR Mode/Subsystem ==
  Bus Creator : BusCreator  Inputs=3
  Bus Creator1 : BusCreator  Inputs=2
  Bus Creator2 : BusCreator  Inputs=2
  Constant : Constant  Value=zeros(12,1)
  Constant1 : Constant  Value=zeros(12,1)
  Constant2 : Constant  Value=zeros(4,1)
  Constant3 : Constant  Value=zeros(4,1)
  Constant4 : Constant  Value=zeros(4,1)
  Fake Panda : Outport
  wires:
  Constant/1 -> Bus Creator1/1  "Distances"
  Constant1/1 -> Bus Creator1/2  "Angles"
  Constant2/1 -> Bus Creator/1  "Color"
  Constant3/1 -> Bus Creator/2  "Probability"
  Constant4/1 -> Bus Creator/3  "idx"
  Bus Creator1/1 -> Bus Creator2/1  "Landmarks"
  Bus Creator/1 -> Bus Creator2/2  "Color data"
  Bus Creator2/1 -> Fake Panda/1  "Lidar Data Input"

== system RobotX_ss_acousticsSingle_Dock_LB_ODOA_T_1024_NewLidarMode/Sensors/1024 Comms New LIDAR Mode/UTC Timer ==
  Start Time : Inport
  MATLAB Function : MATLAB Function  TreatAsAtomicUnit=on
  Real Time : Outport
  wires:
  Start Time/1 -> MATLAB Function/1(inTime)
  MATLAB Function/1(timeOut) -> Real Time/1

== system RobotX_ss_acousticsSingle_Dock_LB_ODOA_T_1024_NewLidarMode/Sensors/1024 Comms New LIDAR Mode/data log ==
  Sensors signal : Inport
  Bus to Vector : BusToVector
  Read : DataStoreRead  DataStoreName=PingPose
  Scope 2 : slrtlib/Displays and Logging/Scope   scopeno=2  scopetype=File  autostart=on  viewmode=Graphical redraw  formatstr='%15.6f'  grid=on  ylimits=[0,0]  nosamples=250  noprepostsamples=0  interleave=1  triggermode=FreeRun  triggersignal=1  trigsignalfromport=off  triggerlevel=0.0  triggerslope=Either  triggerscope=1  triggersample=0  filename=NAL1_<%%%>1.dat  mode=Commit  writesize=512  autorestart=on  dynamicfilemode=on  maxwritefilesize=512*1024^2
  Scope 4 : slrtlib/Displays and Logging/Scope   scopeno=1  scopetype=File  autostart=on  viewmode=Graphical redraw  formatstr='%15.6f'  grid=on  ylimits=[0,0]  nosamples=250  noprepostsamples=0  interleave=1  triggermode=FreeRun  triggersignal=1  trigsignalfromport=off  triggerlevel=0.0  triggerslope=Either  triggerscope=1  triggersample=0  filename=pPos_<%%%>1.dat  mode=Commit  writesize=512  autorestart=on  dynamicfilemode=on  maxwritefilesize=512*1024^2
  wires:
  Sensors signal/1 -> Bus to Vector/1
  Bus to Vector/1 -> Scope 2/1
  Read/1 -> Scope 4/1

== system RobotX_ss_acousticsSingle_Dock_LB_ODOA_T_1024_NewLidarMode/Main FSM/Acoustic Single Point FSM/Acoustics Orient/Output Heirarchy ==
  Data : Inport
  Sensors : Inport  Port=2
  Acoustic Active : Constant
  Bus Creator2 : BusCreator  Inputs=3
  Bus Creator3 : BusCreator  Inputs=3
  Bus Creator5 : BusCreator  Inputs=2
  Constant : Constant
  Constant3 : Constant
  Lidar Mode : Constant
  Outputs : Outport
  wires:
  Sensors/1 -> Bus Creator5/2  "Sensors"
  Bus Creator5/1 -> Outputs/1  "Output Signals"
  Constant/1 -> Bus Creator2/1  "Valid"
  Constant3/1 -> Bus Creator2/2  "Control Mode"
  Data/1 -> Bus Creator2/3  "Data"
  Bus Creator2/1 -> Bus Creator3/1  "Navigation Outputs"
  Acoustic Active/1 -> Bus Creator3/2  "Acoustic Active"
  Lidar Mode/1 -> Bus Creator3/3  "Lidar Mode"
  Bus Creator3/1 -> Bus Creator5/1  "Outputs"

== system RobotX_ss_acousticsSingle_Dock_LB_ODOA_T_1024_NewLidarMode/Main FSM/Acoustic Single Point FSM/Move/Output Reassign ==
  Vaild : Inport
  Data : Inport  Port=2
  Sensors : Inport  Port=3
  Acoustic Active : Constant  Value=0
  Bus Creator2 : BusCreator  Inputs=3
  Bus Creator3 : BusCreator  Inputs=3
  Bus Creator5 : BusCreator  Inputs=2
  Constant3 : Constant  Value=0
  Lidar Mode : Constant  Value=0
  Outputs : Outport
  wires:
  Sensors/1 -> Bus Creator5/2  "Sensors"
  Bus Creator5/1 -> Outputs/1  "Output Signals"
  Vaild/1 -> Bus Creator2/1  "Valid"
  Constant3/1 -> Bus Creator2/2  "Control Mode"
  Data/1 -> Bus Creator2/3  "Data"
  Bus Creator2/1 -> Bus Creator3/1  "Navigation Outputs"
  Acoustic Active/1 -> Bus Creator3/2  "Acoustic Active"
  Lidar Mode/1 -> Bus Creator3/3  "Lidar Mode"
  Bus Creator3/1 -> Bus Creator5/1  "Outputs"

== system RobotX_ss_acousticsSingle_Dock_LB_ODOA_T_1024_NewLidarMode/Main FSM/Acoustic Single Point FSM/Report/Output Heirarchy ==
  Sensors : Inport
  Data : Inport  Port=2
  Acoustic Active : Constant
  Bus Creator2 : BusCreator  Inputs=3
  Bus Creator3 : BusCreator  Inputs=3
  Bus Creator5 : BusCreator  Inputs=2
  Constant : Constant
  Constant3 : Constant
  Lidar Mode : Constant
  Outputs : Outport
  wires:
  Sensors/1 -> Bus Creator5/2  "Sensors"
  Bus Creator5/1 -> Outputs/1  "Output Signals"
  Constant/1 -> Bus Creator2/1  "Valid"
  Constant3/1 -> Bus Creator2/2  "Control Mode"
  Data/1 -> Bus Creator2/3  "Data"
  Bus Creator2/1 -> Bus Creator3/1  "Navigation Outputs"
  Acoustic Active/1 -> Bus Creator3/2  "Acoustic Active"
  Lidar Mode/1 -> Bus Creator3/3  "Lidar Mode"
  Bus Creator3/1 -> Bus Creator5/1  "Outputs"

== system RobotX_ss_acousticsSingle_Dock_LB_ODOA_T_1024_NewLidarMode/Main FSM/Docking/Docking/Output Heirarchy ==
  Data : Inport
  Sensors : Inport  Port=2
  Acoustic Active : Constant  Value=0
  Bus Creator2 : BusCreator  Inputs=3
  Bus Creator3 : BusCreator  Inputs=3
  Bus Creator5 : BusCreator  Inputs=2
  Constant : Constant
  Constant3 : Constant
  Lidar Mode : Constant  Value=2
  Outputs : Outport
  wires:
  Sensors/1 -> Bus Creator5/2  "Sensors"
  Bus Creator5/1 -> Outputs/1  "Output Signals"
  Constant/1 -> Bus Creator2/1  "Valid"
  Constant3/1 -> Bus Creator2/2  "Control Mode"
  Data/1 -> Bus Creator2/3  "Data"
  Bus Creator2/1 -> Bus Creator3/1  "Navigation Outputs"
  Acoustic Active/1 -> Bus Creator3/2  "Acoustic Active"
  Lidar Mode/1 -> Bus Creator3/3  "Lidar Mode"
  Bus Creator3/1 -> Bus Creator5/1  "Outputs"

== system RobotX_ss_acousticsSingle_Dock_LB_ODOA_T_1024_NewLidarMode/Main FSM/Docking/GPS Move/Output Reassign ==
  Vaild : Inport
  Data : Inport  Port=2
  Sensors : Inport  Port=3
  Acoustic Active : Constant  Value=0
  Bus Creator2 : BusCreator  Inputs=3
  Bus Creator3 : BusCreator  Inputs=3
  Bus Creator5 : BusCreator  Inputs=2
  Constant3 : Constant  Value=0
  Lidar Mode : Constant  Value=0
  Outputs : Outport
  wires:
  Sensors/1 -> Bus Creator5/2  "Sensors"
  Bus Creator5/1 -> Outputs/1  "Output Signals"
  Vaild/1 -> Bus Creator2/1  "Valid"
  Constant3/1 -> Bus Creator2/2  "Control Mode"
  Data/1 -> Bus Creator2/3  "Data"
  Bus Creator2/1 -> Bus Creator3/1  "Navigation Outputs"
  Acoustic Active/1 -> Bus Creator3/2  "Acoustic Active"
  Lidar Mode/1 -> Bus Creator3/3  "Lidar Mode"
  Bus Creator3/1 -> Bus Creator5/1  "Outputs"

== system RobotX_ss_acousticsSingle_Dock_LB_ODOA_T_1024_NewLidarMode/Main FSM/Docking/Reverse/Output Heirarchy ==
  Sensors : Inport
  Acoustic Active : Constant  Value=0
  Bus Creator2 : BusCreator  Inputs=3
  Bus Creator3 : BusCreator  Inputs=3
  Bus Creator5 : BusCreator  Inputs=2
  Constant2 : Constant  Value=[-100; -100; zeros(22,1)]
  Constant3 : Constant
  Constant4 : Constant  Value=2
  Lidar Mode : Constant  Value=2
  Outputs : Outport
  wires:
  Sensors/1 -> Bus Creator5/2  "Sensors"
  Bus Creator5/1 -> Outputs/1  "Output Signals"
  Constant3/1 -> Bus Creator2/1  "Valid"
  Constant4/1 -> Bus Creator2/2  "Control Mode"
  Constant2/1 -> Bus Creator2/3  "Data"
  Bus Creator2/1 -> Bus Creator3/1  "Navigation Outputs"
  Acoustic Active/1 -> Bus Creator3/2  "Acoustic Active"
  Lidar Mode/1 -> Bus Creator3/3  "Lidar Mode"
  Bus Creator3/1 -> Bus Creator5/1  "Outputs"

== system RobotX_ss_acousticsSingle_Dock_LB_ODOA_T_1024_NewLidarMode/Main FSM/LightTower/Approach Light Tower/Output Reassign ==
  Vaild : Inport
  Data : Inport  Port=2
  Sensors : Inport  Port=3
  Acoustic Active : Constant  Value=0
  Bus Creator2 : BusCreator  Inputs=3
  Bus Creator3 : BusCreator  Inputs=3
  Bus Creator5 : BusCreator  Inputs=2
  Constant3 : Constant  Value=0
  Lidar Mode : Constant  Value=7
  Outputs : Outport
  wires:
  Sensors/1 -> Bus Creator5/2  "Sensors"
  Bus Creator5/1 -> Outputs/1  "Output Signals"
  Vaild/1 -> Bus Creator2/1  "Valid"
  Constant3/1 -> Bus Creator2/2  "Control Mode"
  Data/1 -> Bus Creator2/3  "Data"
  Bus Creator2/1 -> Bus Creator3/1  "Navigation Outputs"
  Acoustic Active/1 -> Bus Creator3/2  "Acoustic Active"
  Lidar Mode/1 -> Bus Creator3/3  "Lidar Mode"
  Bus Creator3/1 -> Bus Creator5/1  "Outputs"

== system RobotX_ss_acousticsSingle_Dock_LB_ODOA_T_1024_NewLidarMode/Main FSM/LightTower/Go to Field Corner/Output Reassign ==
  Vaild : Inport
  Data : Inport  Port=2
  Sensors : Inport  Port=3
  Acoustic Active : Constant  Value=0
  Bus Creator2 : BusCreator  Inputs=3
  Bus Creator3 : BusCreator  Inputs=3
  Bus Creator5 : BusCreator  Inputs=2
  Constant3 : Constant
  Lidar Mode : Constant  Value=7
  Outputs : Outport
  wires:
  Sensors/1 -> Bus Creator5/2  "Sensors"
  Bus Creator5/1 -> Outputs/1  "Output Signals"
  Vaild/1 -> Bus Creator2/1  "Valid"
  Constant3/1 -> Bus Creator2/2  "Control Mode"
  Data/1 -> Bus Creator2/3  "Data"
  Bus Creator2/1 -> Bus Creator3/1  "Navigation Outputs"
  Acoustic Active/1 -> Bus Creator3/2  "Acoustic Active"
  Lidar Mode/1 -> Bus Creator3/3  "Lidar Mode"
  Bus Creator3/1 -> Bus Creator5/1  "Outputs"

== system RobotX_ss_acousticsSingle_Dock_LB_ODOA_T_1024_NewLidarMode/Main FSM/LightTower/Point Toward Last Known Heading/Output Reassign ==
  Data : Inport
  Sensors : Inport  Port=2
  Acoustic Active : Constant  Value=0
  Bus Creator2 : BusCreator  Inputs=3
  Bus Creator3 : BusCreator  Inputs=3
  Bus Creator5 : BusCreator  Inputs=2
  Constant1 : Constant
  Constant3 : Constant
  Lidar Mode : Constant  Value=7
  Outputs : Outport
  wires:
  Sensors/1 -> Bus Creator5/2  "Sensors"
  Bus Creator5/1 -> Outputs/1  "Output Signals"
  Constant1/1 -> Bus Creator2/1  "Valid"
  Constant3/1 -> Bus Creator2/2  "Control Mode"
  Data/1 -> Bus Creator2/3  "Data"
  Bus Creator2/1 -> Bus Creator3/1  "Navigation Outputs"
  Acoustic Active/1 -> Bus Creator3/2  "Acoustic Active"
  Lidar Mode/1 -> Bus Creator3/3  "Lidar Mode"
  Bus Creator3/1 -> Bus Creator5/1  "Outputs"

== system RobotX_ss_acousticsSingle_Dock_LB_ODOA_T_1024_NewLidarMode/Main FSM/LightTower/Report and Manuever Away/Output Reassign1 ==
  Data : Inport
  Valid : Inport  Port=2
  Sensors : Inport  Port=3
  Acoustic Active : Constant  Value=0
  Bus Creator2 : BusCreator  Inputs=3
  Bus Creator3 : BusCreator  Inputs=3
  Bus Creator5 : BusCreator  Inputs=2
  Constant3 : Constant
  Lidar Mode : Constant  Value=0
  Outputs : Outport
  wires:
  Sensors/1 -> Bus Creator5/2  "Sensors"
  Bus Creator5/1 -> Outputs/1  "Output Signals"
  Valid/1 -> Bus Creator2/1  "Valid"
  Constant3/1 -> Bus Creator2/2  "Control Mode"
  Data/1 -> Bus Creator2/3  "Data"
  Bus Creator2/1 -> Bus Creator3/1  "Navigation Outputs"
  Acoustic Active/1 -> Bus Creator3/2  "Acoustic Active"
  Lidar Mode/1 -> Bus Creator3/3  "Lidar Mode"
  Bus Creator3/1 -> Bus Creator5/1  "Outputs"

== system RobotX_ss_acousticsSingle_Dock_LB_ODOA_T_1024_NewLidarMode/Main FSM/LightTower/Sweep Field/Drive to Point ==
  Sensors : Inport
  Enable : EnablePort
  Bus Selector : BusSelector  OutputSignals=Navigation Message.Pose.X,Navigation Message.Pose.Y,Navigation Message.Pose.Psi,Lidar Data Input.Landmarks.Distances,Lidar Data Input.Landmarks.Angles,Navigation Message.Velocity.u
  Bus Selector1 : BusSelector  OutputSignals=Navigation Message.Pose.X,Navigation Message.Pose.Y,Navigation Message.Pose.Psi
  CalcTimes : MATLAB Function  TreatAsAtomicUnit=on
  Data Store Read : DataStoreRead  DataStoreName=LTSubsetCorners
  Data Store Write : DataStoreWrite  DataStoreName=LTLocationNED
  Data Type Conversion : DataTypeConversion  OutDataTypeStr=double
  Distance to Travel : Constant  Value=5
  GPSMove with Tower Search : MATLAB Function  TreatAsAtomicUnit=on
  MATLAB Function : MATLAB Function  TreatAsAtomicUnit=on
  Output Reassign : Subsystem
  Outputs : Outport
  Finished : Outport  Port=2
  Found LT : Outport  Port=3
  wires:
  GPSMove with Tower Search/1(Finished) -> Data Type Conversion/1
  GPSMove with Tower Search/3(pts) -> CalcTimes/1(pts)
  Data Type Conversion/1 -> Finished/1
  Sensors/1 -> Bus Selector/1, Output Reassign/3(Sensors), Bus Selector1/1
  Bus Selector/1 -> GPSMove with Tower Search/2(X)  "<X>"
  Bus Selector/2 -> GPSMove with Tower Search/3(Y)  "<Y>"
  Bus Selector/3 -> GPSMove with Tower Search/4(Psi)  "<Psi>"
  Bus Selector/6 -> CalcTimes/2(u)  "<u>"
  CalcTimes/1(Data) -> Output Reassign/2(Data)
  Output Reassign/1(Outputs) -> Outputs/1
  GPSMove with Tower Search/2(valid) -> Output Reassign/1(Vaild)
  Bus Selector1/1 -> MATLAB Function/1(X)  "<X>"
  Bus Selector1/2 -> MATLAB Function/2(Y)  "<Y>"
  MATLAB Function/1(GoalNED) -> GPSMove with Tower Search/1(GoalNED)
  Bus Selector1/3 -> MATLAB Function/3(Psi)  "<Psi>"
  Distance to Travel/1 -> MATLAB Function/4(dist)
  Data Store Read/1 -> GPSMove with Tower Search/5(LTsubset)
  Bus Selector/4 -> GPSMove with Tower Search/6(Distances)  "<Distances>"
  Bus Selector/5 -> GPSMove with Tower Search/7(Angles)  "<Angles>"
  GPSMove with Tower Search/4(FoundTower) -> Found LT/1
  GPSMove with Tower Search/5(TowerLoc) -> Data Store Write/1

== system RobotX_ss_acousticsSingle_Dock_LB_ODOA_T_1024_NewLidarMode/Main FSM/LightTower/Sweep Field/Spin, Listen, and Point ==
  Sensors : Inport
  Enable : EnablePort
  Bus Selector : BusSelector  OutputSignals=Navigation Message.Pose.X,Navigation Message.Pose.Y,Navigation Message.Pose.Psi,Lidar Data Input.Landmarks.Distances,Lidar Data Input.Landmarks.Angles
  Data Store Read1 : DataStoreRead  DataStoreName=LTSubsetCorners
  Data Store Write : DataStoreWrite  DialogController=Simulink.DDGSource  DataStoreName=LTLocationNED
  Look for Light Tower : MATLAB Function  TreatAsAtomicUnit=on
  Output Reassign1 : Subsystem
  Total Spin Amount (Deg) : Constant  Value=60
  Outputs : Outport
  Finished : Outport  Port=2
  Found LT : Outport  Port=3
  wires:
  Look for Light Tower/2(Finished) -> Finished/1
  Output Reassign1/1(Outputs) -> Outputs/1
  Look for Light Tower/1(Data) -> Output Reassign1/1(Data)
  Sensors/1 -> Output Reassign1/2(Sensors), Bus Selector/1
  Bus Selector/3 -> Look for Light Tower/4(Psi)  "<Psi>"
  Bus Selector/2 -> Look for Light Tower/3(Y)  "<Y>"
  Bus Selector/5 -> Look for Light Tower/6(Angles)  "<Angles>"
  Bus Selector/1 -> Look for Light Tower/2(X)  "<X>"
  Bus Selector/4 -> Look for Light Tower/5(Distances)  "<Distances>"
  Data Store Read1/1 -> Look for Light Tower/1(subsetCorners)
  Look for Light Tower/3(FoundTower) -> Found LT/1
  Look for Light Tower/4(TowerLoc) -> Data Store Write/1
  Total Spin Amount (Deg)/1 -> Look for Light Tower/7(spinAmount)

== system RobotX_ss_acousticsSingle_Dock_LB_ODOA_T_1024_NewLidarMode/Main FSM/LightTower/Sweep Field/Task Option ==
  note: Acoustic Location Options
      |
      | > 'PingSrch' - assumes it is at the starting
      | GPS point and begins the search spiral/grid
      |
      | >'FindBuoy' - assumes the pinger has been
      | heard for two consecutive samples and
      | begins to search from the current location
      | for the first buoy it sees
      |
      | >'Approach' - approaches the buoy that is
      | in the field of view until it is within .5 to 2
      | meters of the buoy, stops, and stores the
      | buoy properties.
      |
      | >'Report' - Reports the buoy information.
  Acoustic Location : Constant  Value=uint8('Navigate')  SampleTime=.25
  Message Composer : MATLAB Function  TreatAsAtomicUnit=on
  Option : Outport
  wires:
  Acoustic Location/1 -> Message Composer/1(taskStrInit)
  Message Composer/1(taskStrAdj) -> Option/1
